simulink model "firesystem"  (R2020a)
settings: Solver=VariableStepAuto  StartTime=0.0  StopTime=10.0  RelTol=1e-3
libraries: arduinolib x3
settings Model: Creator=pc  LastModifiedBy=pc

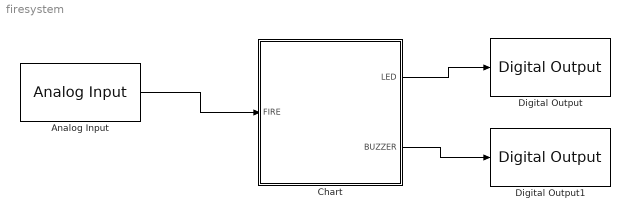
== system firesystem ==
  Analog Input : arduinolib/Analog Input  pinNumber=0  ReadResultsOnly=off  ConversionTriggerSource=Software  ExternalTriggerType=uint32( 0 )  OutputDataType=uint16  EnableConversionCompleteNotify=off  EnableOuputStatus=off  SampleTime=-1  blockPlatform=arduino
  Chart : Stateflow chart  TreatAsAtomicUnit=on
  Digital Output : arduinolib/Digital Output  pinNumber=9  Direction=output  blockPlatform=arduino
  Digital Output1 : arduinolib/Digital Output  pinNumber=5  Direction=output  blockPlatform=arduino
  wires:
  Chart/1(LED) -> Digital Output/1
  Chart/2(BUZZER) -> Digital Output1/1
  Analog Input/1 -> Chart/1(FIRE)

== stateflow chart firesystem/Chart ==
  state FireOn
    LED=1;
    BUZZER=1;
  state FireOff
    LED=1;
    BUZZER=1;
  (default) -> FireOn
  FireOn -> FireOff : [FIRE <= 50]
  FireOff -> FireOn : [FIRE > 50]
  data: LED output; BUZZER output; FIRE input
